simulink library "Radiator_AIV"  (Simulink 8.2)
settings: Solver=ode45  StartTime=0.0  StopTime=10.0  RelTol=1e-3
libraries: carnot x1
settings Model: Creator=lena.frank  LastModifiedBy=drhf

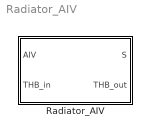
== system Radiator_AIV ==
  Radiator_AIV : Subsystem  mask(radiator){pnom=500, dtnom=40, expo=1.3, mcap=5*4182, ra=0.47, tini=20, lin=10, qua=10}
      mask prompts: pnom "nominal power per unit in W"; dtnom "nominal temperature difference in K"; expo "radiator exponent (> 0)"; mcap "mass * capacity per unit in J/K"; ra "radiative part of heat transfer (0..1)"; tini "initial temperature in degree Celsius"; lin "linear pressure drop dependace of massflow in Pa*s/kg"; qua "quadratic pressure drop dependace of massflow in Pa*s²/kg²"
      mask help: Calculates the power of a radiator according to the nominal power the and the temperaure difference.
      mask init:
      | ra = max(0, min(1, ra));
      | co = 1-ra;
      mask Help: web(['file:///' fullfile(path_carnot('help'),'Radiator.html')],'-helpbrowser')
      mask Display:
      | plot(-20,0,120,90,[20 90 90 20 20],[20 20 70 70 20],[30 30],[25 65],[40 40],[25 65],[50 50],[25 65],[60 60],[25 65],[70 70],[25 65],[80 80],[25 65],[15 20],[25 25],[15 20],[65 65])
      | port_label('input',1,'AIV')
      | port_label('input',2,'THB')
      | port_label('output',1,'[S]')
      | port_label('output',2,'THB')

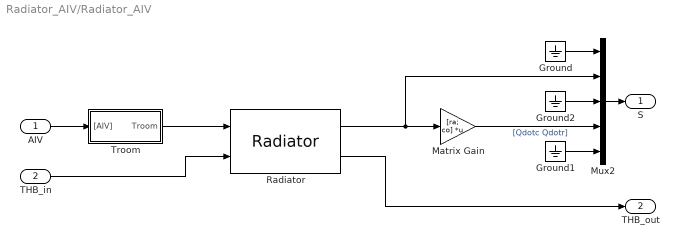
== system Radiator_AIV/Radiator_AIV ==
  AIV : Inport
  THB_in : Inport  Port=2
  Ground : Ground
  Ground1 : Ground
  Ground2 : Ground
  Matrix Gain : Gain  Gain=[ra; co]  Multiplication=Matrix(K*u)  SaturateOnIntegerOverflow=on  OutDataTypeStr=Inherit: Same as input  ParamDataTypeStr=Inherit: Same as input
  Mux2 : Mux  Inputs=[4 1 1 2 5]
  Radiator : carnot/Source/Heat_Exchanger/Radiator  pnom=pnom  dtnom=dtnom  expo=expo  mcap=mcap  tini=tini  lin=lin  qua=qua
  Troom : Subsystem
  S : Outport
  THB_out : Outport  Port=2
  wires:
  Radiator/2 -> THB_out/1
  THB_in/1 -> Radiator/2
  Troom/1(Troom) -> Radiator/1
  AIV/1 -> Troom/1("[AIV]")
  Radiator/1 -> Mux2/2, Matrix Gain/1
  Matrix Gain/1 -> Mux2/4  "[Qdotc Qdotr]"
  Mux2/1 -> S/1
  Ground1/1 -> Mux2/5
  Ground2/1 -> Mux2/3
  Ground/1 -> Mux2/1

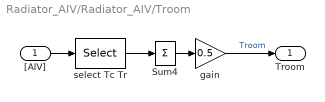
== system Radiator_AIV/Radiator_AIV/Troom ==
  "[AIV]" : Inport
  Sum4 : Sum  Inputs=1  SaturateOnIntegerOverflow=on  InputSameDT=on  OutDataTypeStr=Inherit: Same as first input
  gain : Gain  Gain=0.5  SaturateOnIntegerOverflow=on  OutDataTypeStr=Inherit: Same as input  ParamDataTypeStr=Inherit: Same as input
  select Tc Tr : Selector  InputPortWidth=9  IndexOptions=Index vector (dialog)  Indices=[2 3]  OutputSizes=1
  Troom : Outport
  wires:
  "[AIV]"/1 -> select Tc Tr/1
  gain/1 -> Troom/1  "Troom"
  Sum4/1 -> gain/1
  select Tc Tr/1 -> Sum4/1
